simulink model "recursive_running_sum_2"  (R2014b)
settings: Solver=ode45  StartTime=0.0  StopTime=inf  RelTol=1e-3
undefined symbols (not defined in the file or in its folder): filtk
libraries: dsparch4 x3, simulink x2, dspmlti4 x2, commsynccomp2 x1
settings Model: NumberOfSteps=8192  Creator=Ben  LastModifiedBy=Ben

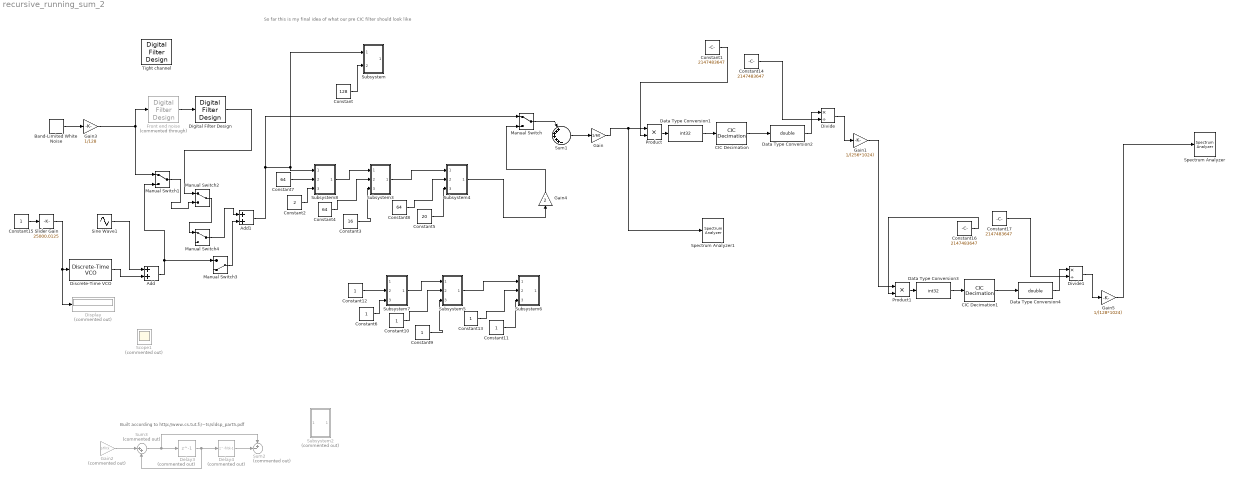
== system recursive_running_sum_2 ==
  note: So far this is my final idea of what our pre CIC filter should look like
  note: Built according to http://www.cs.tut.fi/~ts/sldsp_part5.pdf
  Add : Sum
  Add1 : Sum
  Band-Limited White Noise : simulink/Sources/Band-Limited White Noise  Cov=[0.0001]  Ts=1/250E6  seed=[23341]
  CIC Decimation : dspmlti4/CIC Decimation  filtFrom=Dialog  filtobj=Hm_decim  ftype=Decimator  R=6  M=1  N=8  filterInternals=Full precision  BPS=[16 16 16 16]  FLPS=0  outputWordLength=32  outputFracLength=0  launchFVT=off  framing=Maintain input frame rate  RateOptions=Allow multirate processing
  CIC Decimation1 : dspmlti4/CIC Decimation  filtFrom=Dialog  filtobj=Hm_decim  ftype=Decimator  R=8  M=1  N=8  filterInternals=Full precision  BPS=[16 16 16 16]  FLPS=0  outputWordLength=32  outputFracLength=0  launchFVT=off  framing=Maintain input frame rate  RateOptions=Allow multirate processing
  Constant : Constant  Value=128
  Constant{1,14,16..17} (4 alike) : Constant  Value=2147483647
  Constant{6,9..13} (6 alike) : Constant
  Constant15 : Constant  SampleTime=1/250E6
  Constant2 : Constant  Value=2
  Constant3 : Constant  Value=16
  Constant4 : Constant  Value=64
  Constant5 : Constant  Value=20
  Constant7 : Constant  Value=64
  Constant8 : Constant  Value=64
  Data Type Conversion1 : DataTypeConversion  OutDataTypeStr=int32
  Data Type Conversion2 : DataTypeConversion  OutDataTypeStr=double
  Data Type Conversion3 : DataTypeConversion  OutDataTypeStr=int32
  Data Type Conversion4 : DataTypeConversion  OutDataTypeStr=double
  Delay3 : Delay  Commented=on  DelayLength=1  InitialCondition=0
  Delay4 : Delay  Commented=on  DelayLength=filtk-1  InitialCondition=0
  Digital Filter Design : dsparch4/Digital Filter Design  mwdsp_browser_bugfix_var=off
  Discrete-Time VCO : commsynccomp2/Discrete-Time VCO  Ac=4  Fc=0  Kc=10  Ph=0  ts=1/250E6
  Display : Display  Commented=on
  Divide : Product  Inputs=*/
  Divide1 : Product  Inputs=*/
  "Front end noise " : dsparch4/Digital Filter Design  Commented=through  mwdsp_browser_bugfix_var=off
  Gain : Gain  Gain=1/60
  Gain1 : Gain  Gain=1/(256*1024)
  Gain2 : Gain  Commented=on  Gain=1/filtk
  Gain3 : Gain  Gain=1/128
  Gain4 : Gain  Gain=2
  Gain5 : Gain  Gain=1/(128*1024)
  Manual Switch{,1..2,4} (4 alike) : ManualSwitch
  Manual Switch3 : ManualSwitch  CurrentSetting=0
  Product : Product
  Product1 : Product
  Scope1 : Scope  Commented=on
      settings: TimeRange=0.0001  YMin=-1  YMax=1  MaxDataPoints=50000
  Sine Wave1 : Sin  Amplitude=0  Frequency=1E6*pi*2  SampleTime=1/250E6
  Slider Gain : simulink/Math Operations/Slider Gain  low=0  gain=25000.0125  high=25000001.25
  Spectrum Analyzer : SpectrumAnalyzer
  Spectrum Analyzer1 : SpectrumAnalyzer
  Subsystem : Subsystem
  Subsystem2 : Subsystem  Commented=on
  Subsystem3 : Subsystem
  Subsystem4 : Subsystem
  Subsystem5 : Subsystem
  Subsystem6 : Subsystem
  Subsystem7 : Subsystem
  Subsystem8 : Subsystem
  Sum1 : Sum  Inputs=|++++++-
  Sum2 : Sum  Commented=on  Inputs=+-|
  Sum3 : Sum  Commented=on  Inputs=|++
  Tight channel : dsparch4/Digital Filter Design  mwdsp_browser_bugfix_var=off
  wires:
  Constant15/1 -> Slider Gain/1
  Gain2/1 -> Sum3/1
  Sum3/1 -> Sum2/1, Delay3/1
  Delay3/1 -> Delay4/1, Sum3/2
  Delay4/1 -> Sum2/2
  Constant/1 -> Subsystem/2(In2)
  Constant7/1 -> Subsystem8/2(In2)
  Subsystem8/1(Out1) -> Subsystem3/1(In1)
  Sum1/1 -> Gain/1
  Band-Limited White Noise/1 -> Gain3/1
  Constant2/1 -> Subsystem8/3(In3)
  Constant4/1 -> Subsystem3/2(In2)
  Constant3/1 -> Subsystem3/3(In3)
  Constant8/1 -> Subsystem4/2(In2)
  Constant5/1 -> Subsystem4/3(In3)
  Subsystem3/1(Out1) -> Subsystem4/1(In1)
  Constant12/1 -> Subsystem7/2(In2)
  Subsystem7/1(Out1) -> Subsystem5/1(In1)
  Constant6/1 -> Subsystem7/3(In3)
  Constant10/1 -> Subsystem5/2(In2)
  Constant9/1 -> Subsystem5/3(In3)
  Constant13/1 -> Subsystem6/2(In2)
  Constant11/1 -> Subsystem6/3(In3)
  Subsystem5/1(Out1) -> Subsystem6/1(In1)
  Manual Switch/1 -> Sum1/1
  Constant1/1 -> Product/2
  Gain/1 -> Spectrum Analyzer1/1, Product/1
  Product/1 -> Data Type Conversion1/1
  Data Type Conversion1/1 -> CIC Decimation/1
  Data Type Conversion2/1 -> Divide/1
  Manual Switch1/1 -> Manual Switch2/2
  Constant14/1 -> Divide/2
  Manual Switch2/1 -> Manual Switch4/1
  Digital Filter Design/1 -> Manual Switch2/1
  "Front end noise "/1 -> Digital Filter Design/1
  Sine Wave1/1 -> Add/1
  Add/1 -> Manual Switch1/2, Manual Switch3/1
  Discrete-Time VCO/1 -> Add/2
  Slider Gain/1 -> Display/1, Discrete-Time VCO/1
  Divide/1 -> Gain1/1
  Add1/1 -> Manual Switch/1, Subsystem8/1(In1), Subsystem/1(In1)
  CIC Decimation/1 -> Data Type Conversion2/1
  Gain3/1 -> Manual Switch1/1, "Front end noise "/1
  Manual Switch3/1 -> Add1/2
  Manual Switch4/1 -> Add1/1
  Gain4/1 -> Manual Switch/2
  Subsystem4/1(Out1) -> Gain4/1
  Constant16/1 -> Product1/2
  Product1/1 -> Data Type Conversion3/1
  Data Type Conversion3/1 -> CIC Decimation1/1
  Data Type Conversion4/1 -> Divide1/1
  Constant17/1 -> Divide1/2
  Divide1/1 -> Gain5/1
  Gain5/1 -> Spectrum Analyzer/1
  CIC Decimation1/1 -> Data Type Conversion4/1
  Gain1/1 -> Product1/1

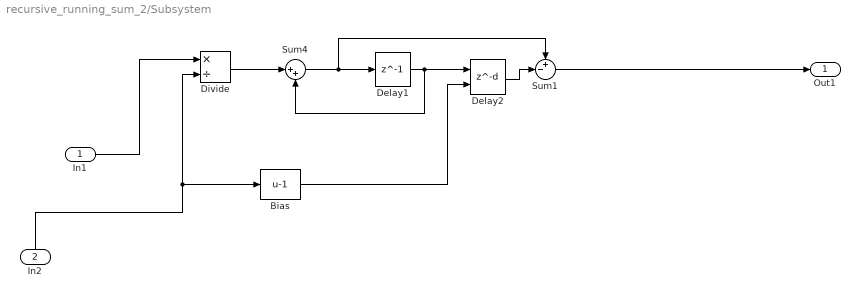
== system recursive_running_sum_2/Subsystem ==
  In1 : Inport
  In2 : Inport  Port=2
  Bias : Bias  Bias=-1
  Delay1 : Delay  DelayLength=1  InitialCondition=0
  Delay2 : Delay  DelayLengthSource=Input port  DelayLength=filtk-1  InitialCondition=0
      settings: InputPortMap=u0,p1
  Divide : Product  Inputs=*/
  Sum1 : Sum  Inputs=+-|
  Sum4 : Sum  Inputs=|++
  Out1 : Outport
  wires:
  Sum4/1 -> Sum1/1, Delay1/1
  Delay1/1 -> Delay2/1, Sum4/2
  Delay2/1 -> Sum1/2
  Sum1/1 -> Out1/1
  In1/1 -> Divide/1
  Divide/1 -> Sum4/1
  Bias/1 -> Delay2/2
  In2/1 -> Divide/2, Bias/1

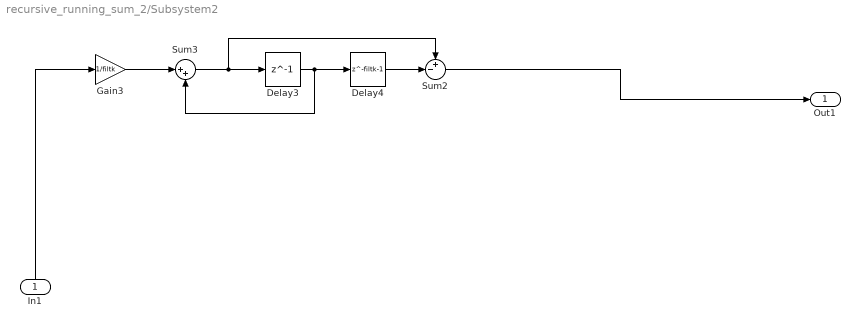
== system recursive_running_sum_2/Subsystem2 ==
  In1 : Inport
  Delay3 : Delay  DelayLength=1  InitialCondition=0
  Delay4 : Delay  DelayLength=filtk-1  InitialCondition=0
  Gain3 : Gain  Gain=1/filtk
  Sum2 : Sum  Inputs=+-|
  Sum3 : Sum  Inputs=|++
  Out1 : Outport
  wires:
  Delay3/1 -> Delay4/1, Sum3/2
  Sum3/1 -> Sum2/1, Delay3/1
  Delay4/1 -> Sum2/2
  Gain3/1 -> Sum3/1
  Sum2/1 -> Out1/1
  In1/1 -> Gain3/1

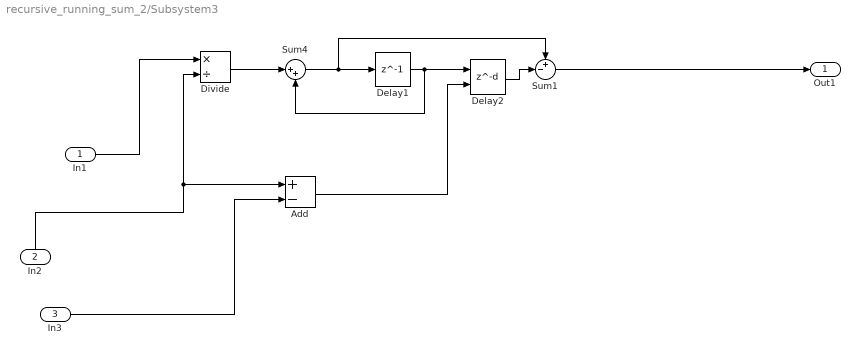
== system recursive_running_sum_2/Subsystem3 ==
  In1 : Inport
  In2 : Inport  Port=2
  In3 : Inport  Port=3
  Add : Sum  Inputs=+-
  Delay1 : Delay  DelayLength=1  InitialCondition=0
  Delay2 : Delay  DelayLengthSource=Input port  DelayLength=filtk-1  InitialCondition=0
      settings: InputPortMap=u0,p1
  Divide : Product  Inputs=*/
  Sum1 : Sum  Inputs=+-|
  Sum4 : Sum  Inputs=|++
  Out1 : Outport
  wires:
  Sum4/1 -> Sum1/1, Delay1/1
  Delay1/1 -> Delay2/1, Sum4/2
  Delay2/1 -> Sum1/2
  Sum1/1 -> Out1/1
  In1/1 -> Divide/1
  Divide/1 -> Sum4/1
  Add/1 -> Delay2/2
  In2/1 -> Divide/2, Add/1
  In3/1 -> Add/2

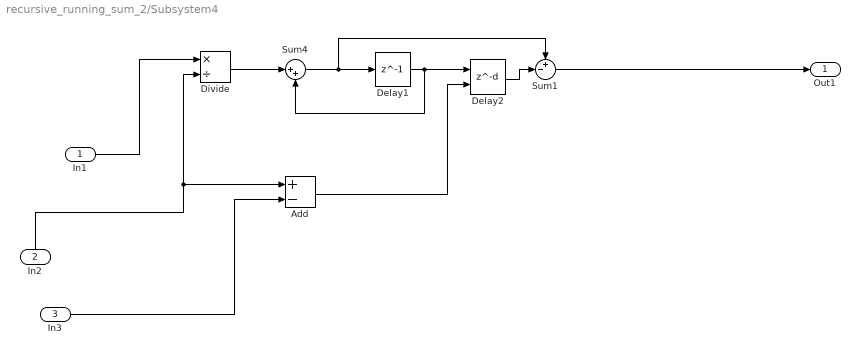
== system recursive_running_sum_2/Subsystem4 ==
  In1 : Inport
  In2 : Inport  Port=2
  In3 : Inport  Port=3
  Add : Sum  Inputs=+-
  Delay1 : Delay  DelayLength=1  InitialCondition=0
  Delay2 : Delay  DelayLengthSource=Input port  DelayLength=filtk-1  InitialCondition=0
      settings: InputPortMap=u0,p1
  Divide : Product  Inputs=*/
  Sum1 : Sum  Inputs=+-|
  Sum4 : Sum  Inputs=|++
  Out1 : Outport
  wires:
  Sum4/1 -> Sum1/1, Delay1/1
  Delay1/1 -> Delay2/1, Sum4/2
  Delay2/1 -> Sum1/2
  Sum1/1 -> Out1/1
  In1/1 -> Divide/1
  Divide/1 -> Sum4/1
  Add/1 -> Delay2/2
  In2/1 -> Divide/2, Add/1
  In3/1 -> Add/2

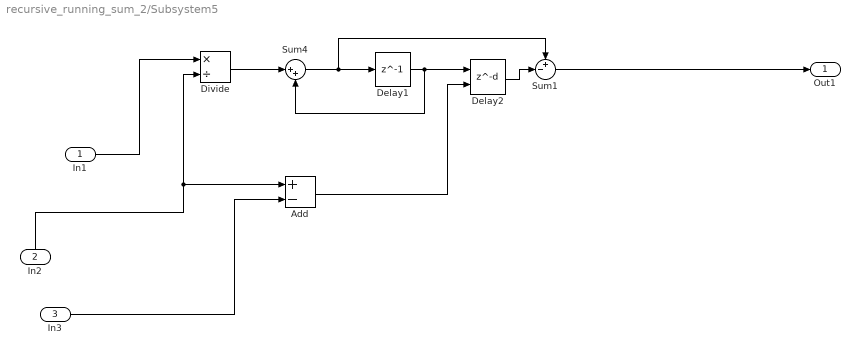
== system recursive_running_sum_2/Subsystem5 ==
  In1 : Inport
  In2 : Inport  Port=2
  In3 : Inport  Port=3
  Add : Sum  Inputs=+-
  Delay1 : Delay  DelayLength=1  InitialCondition=0
  Delay2 : Delay  DelayLengthSource=Input port  DelayLength=filtk-1  InitialCondition=0
      settings: InputPortMap=u0,p1
  Divide : Product  Inputs=*/
  Sum1 : Sum  Inputs=+-|
  Sum4 : Sum  Inputs=|++
  Out1 : Outport
  wires:
  Sum4/1 -> Sum1/1, Delay1/1
  Delay1/1 -> Delay2/1, Sum4/2
  Delay2/1 -> Sum1/2
  Sum1/1 -> Out1/1
  In1/1 -> Divide/1
  Divide/1 -> Sum4/1
  Add/1 -> Delay2/2
  In2/1 -> Divide/2, Add/1
  In3/1 -> Add/2

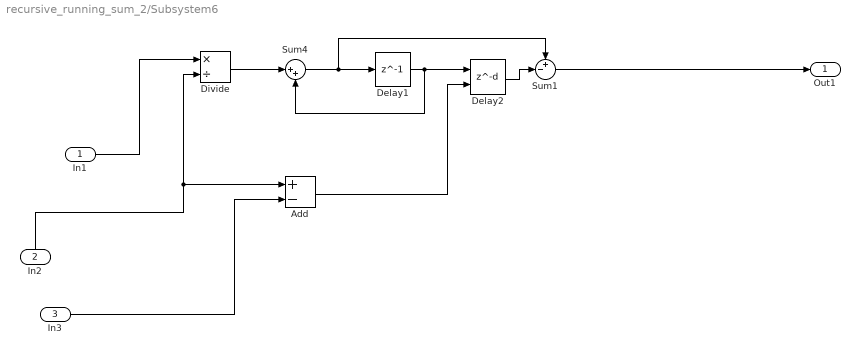
== system recursive_running_sum_2/Subsystem6 ==
  In1 : Inport
  In2 : Inport  Port=2
  In3 : Inport  Port=3
  Add : Sum  Inputs=+-
  Delay1 : Delay  DelayLength=1  InitialCondition=0
  Delay2 : Delay  DelayLengthSource=Input port  DelayLength=filtk-1  InitialCondition=0
      settings: InputPortMap=u0,p1
  Divide : Product  Inputs=*/
  Sum1 : Sum  Inputs=+-|
  Sum4 : Sum  Inputs=|++
  Out1 : Outport
  wires:
  Sum4/1 -> Sum1/1, Delay1/1
  Delay1/1 -> Delay2/1, Sum4/2
  Delay2/1 -> Sum1/2
  Sum1/1 -> Out1/1
  In1/1 -> Divide/1
  Divide/1 -> Sum4/1
  Add/1 -> Delay2/2
  In2/1 -> Divide/2, Add/1
  In3/1 -> Add/2

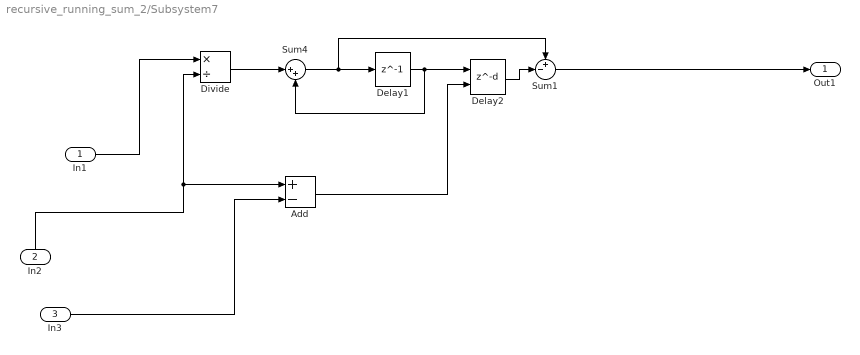
== system recursive_running_sum_2/Subsystem7 ==
  In1 : Inport
  In2 : Inport  Port=2
  In3 : Inport  Port=3
  Add : Sum  Inputs=+-
  Delay1 : Delay  DelayLength=1  InitialCondition=0
  Delay2 : Delay  DelayLengthSource=Input port  DelayLength=filtk-1  InitialCondition=0
      settings: InputPortMap=u0,p1
  Divide : Product  Inputs=*/
  Sum1 : Sum  Inputs=+-|
  Sum4 : Sum  Inputs=|++
  Out1 : Outport
  wires:
  Sum4/1 -> Sum1/1, Delay1/1
  Delay1/1 -> Delay2/1, Sum4/2
  Delay2/1 -> Sum1/2
  Sum1/1 -> Out1/1
  In1/1 -> Divide/1
  Divide/1 -> Sum4/1
  Add/1 -> Delay2/2
  In2/1 -> Divide/2, Add/1
  In3/1 -> Add/2

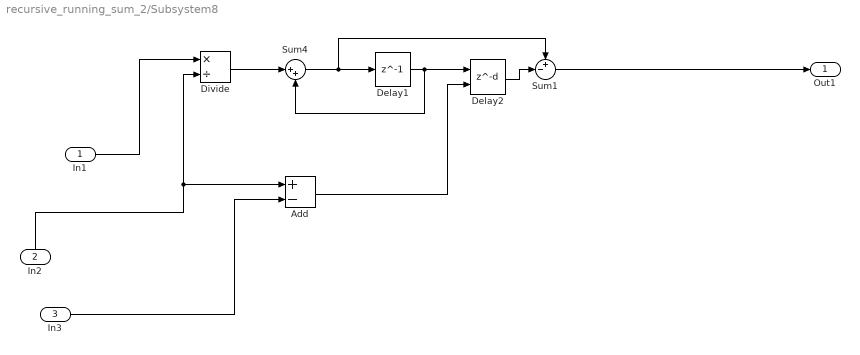
== system recursive_running_sum_2/Subsystem8 ==
  In1 : Inport
  In2 : Inport  Port=2
  In3 : Inport  Port=3
  Add : Sum  Inputs=+-
  Delay1 : Delay  DelayLength=1  InitialCondition=0
  Delay2 : Delay  DelayLengthSource=Input port  DelayLength=filtk-1  InitialCondition=0
      settings: InputPortMap=u0,p1
  Divide : Product  Inputs=*/
  Sum1 : Sum  Inputs=+-|
  Sum4 : Sum  Inputs=|++
  Out1 : Outport
  wires:
  Sum4/1 -> Sum1/1, Delay1/1
  Delay1/1 -> Delay2/1, Sum4/2
  Delay2/1 -> Sum1/2
  Sum1/1 -> Out1/1
  In1/1 -> Divide/1
  Divide/1 -> Sum4/1
  Add/1 -> Delay2/2
  In2/1 -> Divide/2, Add/1
  In3/1 -> Add/2
